simulink model "test_matlab_PV_array_RT_20us"  (Simulink 8.5)
settings: Solver=ode3  StartTime=0.0  StopTime=10  FixedStep=20e-6  RelTol=1e-3
undefined symbols (not defined in the file): another_event_name, Ion, Lithium, my_event_name, sigbuilder_block
libraries: powerlib x8, rtlab x3, artemis x1, electricdrivelib x1, re_lib x1, powerlib_meascontrol x1
settings Model: ARTEMISmethode_block_infos=$$__separator__$$test_matlab_PV_array_RT_20us/ARTEMIS Guide$$__separator__$$  Creator=farhanm  LastModifiedBy=alsetlab
settings DebuggingCC: AlgebraicLoopMsg=error  SolverPrmCheckMsg=warning  FcnCallInpInsideContextMsg=UseLocalSettings

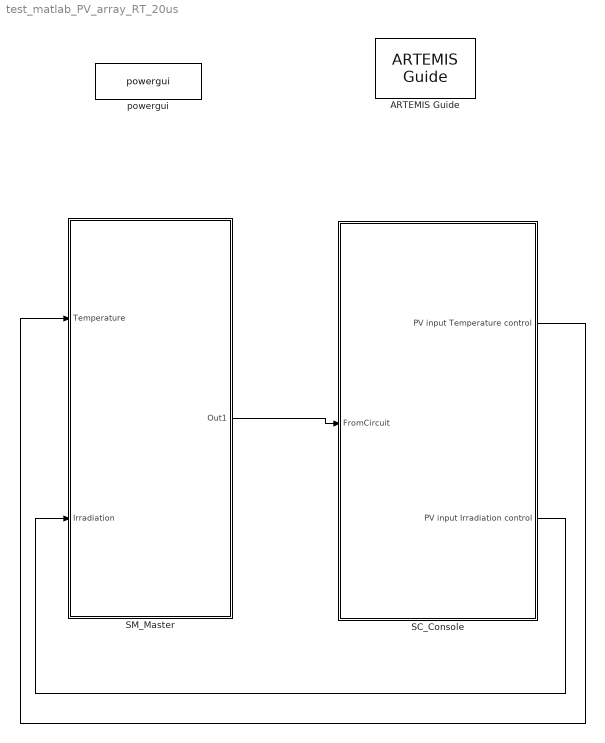
== system test_matlab_PV_array_RT_20us ==
  ARTEMIS Guide : artemis/ARTEMIS/ARTEMIS Guide  Tag=FTSSmethode_opal_4hx0r99  Description=5.0_z1  lock=on  Ts=20e-6  opt=art5  dyna=off  nb_perm=4  RT_fullcomp=off  ssn=on  ssn_itvc=off  ssn_ivic=off  ssn_ext=off  ssn_solver=Art5  ssn_impulse=off  ssn_quasimpulse=off  ssn_impulse_loop=2  paraExtinctionThy=off  Thy_Impulse=on  dtc=Off  dtc_opt=normal  ao=on  simtype=off  ct_mac=off  lin_mov=off  lsp=[0.001 2]  spike_skip=Disabled  dtc_extra=1  dtc_sws=normal  dtc_pied=0.5  SPSRulesBlock=SPSRules  tre=on  ctmm=off  LF=off  dpl_type=ARTEMiS DPL  rlc_type=off  custom_type=off  para=on  ssn_ImpulseLoopBlockedStateUpdate=2  ssn_mov_iter_number=5  ssn_switch_iter_number=5  ssn_nib_type_verify=on  ssn_use_lu=on  ssn_use_ldlt=off
  SC_Console : Subsystem
  SM_Master : Subsystem
  powergui : powerlib/powergui  Priority=1  SimulationMode=Discrete  SolverType=Tustin  SampleTime=20e-6  frequency=60  SPID=off  DisableSnubberDevices=off  DisableRonSwitches=off  DisableVfSwitches=off  SwTol=0  DisplayEquations=off  Interpol=off  methode=off  Ts=100  FunctionMessages=off  echomessages=off  HookPort=off  EnableUseOfTLC=off  x0status=blocks  frequencyindice=0  Pbase=0.5e6  ErrMax=1e-4  Iterations=50  UnitsV=kV  UnitsW=MW  buscounter=0  RestoreLinks=warning  ResistiveCurrentMeasurement=off  Frange=[0:2:500]  Ylog=off  Xlog=on  ShowGrid=off  save=off  variable=ZData  structure=0  ZoomFFT=off  StartTime=0.0  cycles=1  DisplayStyle=1  fundamental=60  FreqAxis=off  MaxFrequency=1000  frequencyindicesteady=1  RmsSteady=1  display=off
  wires:
  SC_Console/1(" PV input Temperature control") -> SM_Master/1(Temperature)
  SC_Console/2(PV input Irradiation control) -> SM_Master/2(Irradiation)
  SM_Master/1(Out1) -> SC_Console/1(FromCircuit)

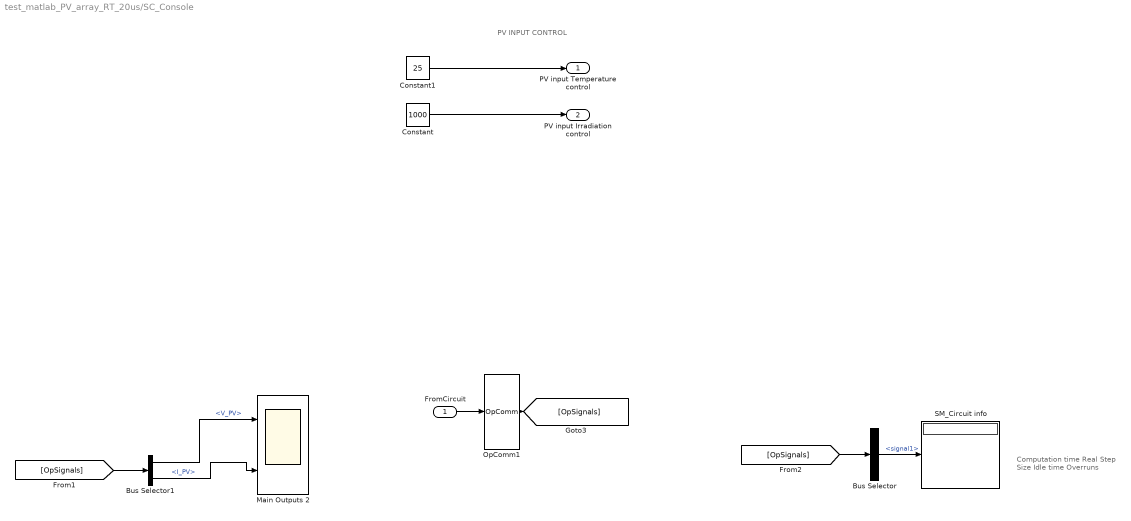
== system test_matlab_PV_array_RT_20us/SC_Console ==
  note: PV INPUT CONTROL
  note: Computation time
      | Real Step Size
      | Idle time
      | Overruns
  FromCircuit : Inport
  Bus Selector : BusSelector  OutputSignals=signal1
  Bus Selector1 : BusSelector  OutputSignals=V_PV,I_PV
  Constant : Constant  Value=1000
  Constant1 : Constant  Value=25
  Main Outputs 2 : Scope  NumInputPorts=2
      settings: TimeRange=10  YMin=0~741.55  YMax=900~742.2
  OpComm1 : rtlab/OpComm  nbport=1  groupe_acq=1  subsys_rate=0  st=0  Synchronization=on  Interpolation=on  Threshold=1  Missed_Data=off  Sim_Time=off  Samples=off  dynSigOut=off  from_console=0  warning_done=off  writeOpCommFile=off  Offset=off
  SM_Circuit info : Display
  " PV input Temperature control" : Outport
  PV input Irradiation control : Outport  Port=2
  wires:
  Constant1/1 -> " PV input Temperature control"/1
  Constant/1 -> PV input Irradiation control/1
  Bus Selector/1 -> SM_Circuit info/1  "<signal1>"
  [OpSignals] -> Bus Selector/1
  OpComm1/1 -> [OpSignals]
  FromCircuit/1 -> OpComm1/1
  Bus Selector1/1 -> Main Outputs 2/1  "<V_PV>"
  Bus Selector1/2 -> Main Outputs 2/2  "<I_PV>"
  [OpSignals] -> Bus Selector1/1

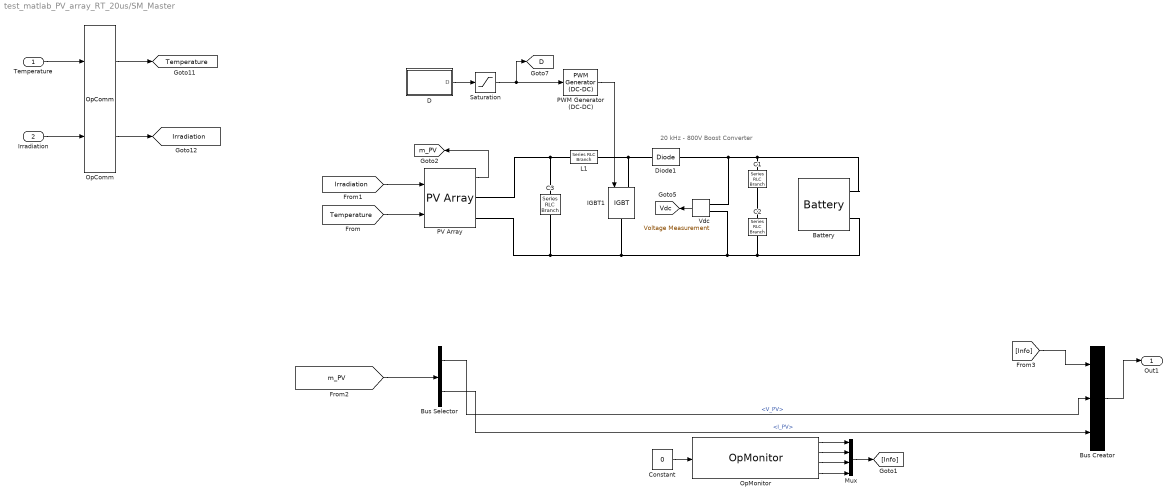
== system test_matlab_PV_array_RT_20us/SM_Master ==
  note: 20 kHz - 800V
      | Boost Converter
  Temperature : Inport
  Irradiation : Inport  Port=2
  Battery : electricdrivelib/Extra Sources/Battery  BatType=Lithium-Ion  ShowDetailedParameters=off  NomV=800  NomQ=1000  SOC=10  PresetModel=on  MaxQ=1000  FullV=931.1897  Dis_rate=434.7826  R=0.008  Normal_OP=904.3478  expZone="[864.3087      49.13043]"  current=[6.5 13 32.5]  Units=Time  Batt_Tr=30
  Bus Creator : BusCreator  Inputs=3
  Bus Selector : BusSelector  OutputSignals=V_PV,I_PV
  C1 : powerlib/Elements/Series RLC Branch  LConnTagsString=__new0  RConnTagsString=__new0  BranchType=C  Resistance=1.0  Inductance=1.0  SetiL0=off  InitialCurrent=0  Capacitance=12000e-06  Setx0=off  InitialVoltage=0  Measurements=None
  C2 : powerlib/Elements/Series RLC Branch  LConnTagsString=__new0  RConnTagsString=__new0  BranchType=C  Resistance=1.0  Inductance=1.0  SetiL0=off  InitialCurrent=0  Capacitance=12000e-06  Setx0=off  InitialVoltage=0  Measurements=None
  C3 : powerlib/Elements/Series RLC Branch  LConnTagsString=__new0  RConnTagsString=__new0  BranchType=C  Resistance=1.0  Inductance=1.0  SetiL0=off  InitialCurrent=0  Capacitance=100e-6  Setx0=off  InitialVoltage=0  Measurements=Branch voltage
  Constant : Constant  Value=0
  D : Subsystem  Tag=STV Subsys  LoadFcn=sigbuilder_block('load');  StartFcn=sigbuilder_block('start');  StopFcn=sigbuilder_block('stop');  ClipboardFcn=sigbuilder_block('clipboard');  mask(Sigbuilder block){}
      mask help: Sigbuilder GUI
      mask init:
      | if ~strcmp(get_param(bdroot(gcbh),'SimulationStatus'),'stopped') tuvar = sigbuilder_block('maskInit'); end
      settings: CopyFcn=sigbuilder_block('copy');  DeleteFcn=sigbuilder_block('delete');  ModelCloseFcn=sigbuilder_block('modelClose');  PreSaveFcn=sigbuilder_block('preSave');  PauseFcn=sigbuilder_block('pause')  ContinueFcn=sigbuilder_block('continue')  NameChangeFcn=sigbuilder_block('namechange');  OpenFcn=sigbuilder_block('open',[6 30 1012.5 446.25 ]);  CloseFcn=sigbuilder_block('close');
      mask Display: plot(0,0,100,100,[10,10,40,40,10],[80,20,20,80,80],[40,10],[50,50], [40,27,10],[65,72,56],[40,25,25,10],[28,28,43,43]);
  Diode1 : powerlib/Power Electronics/Diode  Ron=1e-4  Lon=0  Vf=0  IC=0  UseSnubber=off  Rs=inf  Cs=inf  Measurements=off
  IGBT1 : powerlib/Power Electronics/IGBT  Ron=0.001  Lon=0  Vf=0  Tf=0  Tt=0  IC=0  Rs=1e5  Cs=inf  Measurements=off
  L1 : powerlib/Elements/Series RLC Branch  LConnTagsString=__new0  RConnTagsString=__new0  BranchType=RL  Resistance=0.005  Inductance=5e-3  SetiL0=off  InitialCurrent=0  Capacitance=1e-6  Setx0=off  InitialVoltage=0  Measurements=None
  Mux : Mux
  OpComm : rtlab/OpComm  nbport=2  groupe_acq=1  subsys_rate=20e-6  st=0  Synchronization=on  Interpolation=on  Threshold=1.0  Missed_Data=off  Sim_Time=off  Samples=off  dynSigOut=off  from_console=1  warning_done=off  writeOpCommFile=off  Offset=off
  OpMonitor : rtlab/Monitoring/OpMonitor  compute_time=on  real_step=on  idle_time=on  nb_overruns=on  user_time=off  user_name=my_event_name,another_event_name
  PV Array : re_lib/Solar/PV Array  Npar=140  Nser=20  PlotType=array @ 1000 W/m2 & specified temperatures  S_vec="[ 1000  250 ]"  Temp_C_vec="[0 25 50  ]"  ModuleName=User-defined  PlotWhenSelected=off  Pm=160.3  Ncell=40  Voc=43.8  Isc=5  Vm=35  Im=4.58  beta_Voc_pc=-0.1  alpha_Isc_pc=0.00002  beta_Voc=-0.0438  alpha_Isc=1e-06  IL=4.9966  I0=9.5035e-17  nI=1.1086  Rsh=171.9413  Rs=1.0904  BAL=on  Tc=Tc  Tfilter=5e-5
  PWM Generator (DC-DC) : powerlib_meascontrol/Pulse & Signal Generators/PWM Generator (DC-DC)  Fsw=20000  Ts=20e-06
  Saturation : Saturate  UpperLimit=0.8  LowerLimit=0.2
  "Vdc " : powerlib/Measurements/Voltage Measurement  Tag=PoWeRsYsTeMmEaSuReMeNt  PhasorSimulation=off  OutputType=Magnitude  PSBequivalent=0
  Out1 : Outport
  tag scope: D=global, Irradiation=global, Temperature=global, Vdc=global, m_PV=global
  wires:
  Temperature/1 -> OpComm/1
  Irradiation/1 -> OpComm/2
  OpComm/1 -> [Temperature]
  OpComm/2 -> [Irradiation]
  [m_PV] -> Bus Selector/1
  Bus Selector/2 -> Bus Creator/3  "<I_PV>"
  Bus Selector/1 -> Bus Creator/2  "<V_PV>"
  PV Array/1 -> [m_PV]
  "Vdc "/1 -> [Vdc]
  Saturation/1 -> PWM Generator (DC-DC)/1, [D]
  D/1(D) -> Saturation/1
  PWM Generator (DC-DC)/1 -> IGBT1/1
  [Temperature] -> PV Array/2
  [Irradiation] -> PV Array/1
  Constant/1 -> OpMonitor/1
  Mux/1 -> [Info]
  OpMonitor/2 -> Mux/2
  OpMonitor/3 -> Mux/3
  OpMonitor/4 -> Mux/4
  OpMonitor/1 -> Mux/1
  [Info] -> Bus Creator/1
  Bus Creator/1 -> Out1/1
  connections:
  "Vdc "/LConn1 -- Battery/LConn1 -- C1/LConn1 -- Diode1/RConn1
  Diode1/LConn1 -- IGBT1/LConn1 -- L1/RConn1
  "Vdc "/LConn2 -- IGBT1/RConn1 -- PV Array/RConn2 -- C3/RConn1 -- C2/RConn1 -- Battery/LConn2
  C3/LConn1 -- L1/LConn1 -- PV Array/RConn1
  C2/LConn1 -- C1/RConn1

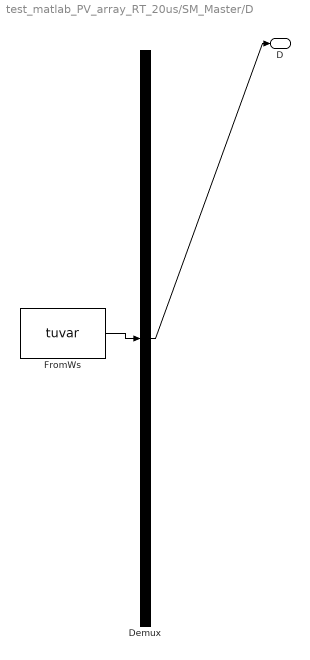
== system test_matlab_PV_array_RT_20us/SM_Master/D ==
  Demux : Demux  Tag=STV Demux  Outputs=1
  FromWs : FromWorkspace  Tag=STV FromWs  VariableName=tuvar  SampleTime=0  SigBuilderData=DataTag0  VnvData=DataTag1
      SigBuilderData=|
      | common.afterFinalStr = 'Extrapolate'
      | common.sampleTime = '0'
      | dataSet(1).timeRange = [0 2]
      | dataSet(1).name = 'Constant Irradiance'
      | dataSet(2).timeRange = [0 2]
      | dataSet(2).name = 'Step Irradiance'
      | dataSet(3).timeRange = [0 3]
      | dataSet(3).name = 'Ramp-up/down Irradiance'
      | sbobj.Groups(1).Name = 'Constant Irradiance'
      | sbobj.Groups(1).Signals.Name = 'D'
      | sbobj.Groups(1).Signals.XData = [0 1.2 1.2 1.8 1.8 3]
      | sbobj.Groups(1).Signals.YData = [0 0 1 1 0 0]
      | sbobj.Groups(1).TimeRange = [0 3]
      | sbobj.Groups(2).Name = 'Step Irradiance'
      | sbobj.Groups(2).Signals.Name = 'D'
      | sbobj.Groups(2).Signals.XData = [0 1.2 1.2 1.8 1.8 3]
      | sbobj.Groups(2).Signals.YData = [0 0 1 1 0 0]
      | sbobj.Groups(2).TimeRange = [0 3]
      | sbobj.Groups(3).Name = 'Ramp-up/down Irradiance'
      | sbobj.Groups(3).Signals.Name = 'D'
      | sbobj.Groups(3).Signals.XData = [0 0.4 0.7 0.8 0.8 3]
      | sbobj.Groups(3).Signals.YData = [0.4 0.4 0.5 0.5 0.45 0.45]
      | sbobj.Groups(3).TimeRange = [0 3]
  D : Outport  Tag=STV Outport
  wires:
  FromWs/1 -> Demux/1
  Demux/1 -> D/1
